simulink model "hw3Q3_model"  (R2021a)
settings: Solver=VariableStepAuto  StartTime=0.0  StopTime=10.0  RelTol=1e-3
values from neighbouring files (symbols this model uses):
  k1 = k1_list(i)    [hw3Q3.m]
  k2 = k2_list(i)    [hw3Q3.m]
settings Model: Creator=kaiyu  LastModifiedBy=kaiyu

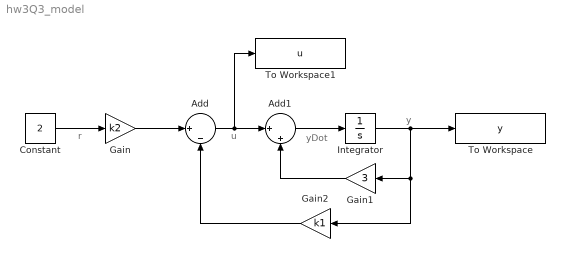
== system hw3Q3_model ==
  note: yDot
  note: y
  note: u
  note: r
  Add : Sum  Inputs=||+|-
  Add1 : Sum  Inputs=||+|+
  Constant : Constant  Value=2
  Gain : Gain  Gain=k2
  Gain1 : Gain  Gain=3
  Gain2 : Gain  Gain=k1
  Integrator : Integrator  InitialCondition=-1
  To Workspace : ToWorkspace  VariableName=y  SaveFormat=Timeseries  SampleTime=-1
  To Workspace1 : ToWorkspace  VariableName=u  SaveFormat=Timeseries  SampleTime=-1
  wires:
  Add/1 -> To Workspace1/1, Add1/1
  Gain/1 -> Add/1
  Add1/1 -> Integrator/1
  Integrator/1 -> Gain2/1, Gain1/1, To Workspace/1
  Gain1/1 -> Add1/2
  Gain2/1 -> Add/2
  Constant/1 -> Gain/1
